simulink model "stumbler_simulation"  (R2024b)
settings: Solver=ode45  StartTime=0.0  StopTime=0.75  RelTol=1e-3  EnableMultiTasking=on
StopFcn:
  | plot_stumbler
settings Model: Creator=Marleen  LastModifiedBy=vijay
settings SolverCC: AlgebraicLoopSolver=TrustRegion
settings DataIOCC: LimitDataPoints=on  SaveFormat=Array  SignalLoggingSaveFormat=ModelDataLogs  ReturnWorkspaceOutputs=off
settings OptimizationCC: InitFltsAndDblsToZero=on  LifeSpan=inf
settings DebuggingCC: SaveWithParameterizedLinksMsg=none  UnderspecifiedInitializationDetection=Classic  MergeDetectMultiDrivingBlocksExec=none  SignalResolutionControl=TryResolveAllWithWarning  SolverPrmCheckMsg=warning  MultiTaskDSMMsg=warning  MultiTaskCondExecSysMsg=none  FcnCallInpInsideContextMsg=warning  UnconnectedInputMsg=warning  UnconnectedOutputMsg=warning  UnconnectedLineMsg=warning  SFUnexpectedBacktrackingDiag=warning  SFNoUnconditionalDefaultTransitionDiag=warning  SFExecutionAtInitializationDiag=none  ArithmeticOperatorsInVariantConditions=warning
settings HardwareCC: ProdBitPerPointer=32  ProdBitPerSizeT=32  ProdBitPerPtrDiffT=32  ProdLargestAtomicFloat=None  ProdIntDivRoundTo=Undefined  ProdEndianess=Unspecified  ProdWordSize=32  ProdHWDeviceType=32-bit Generic
settings ModelReferenceCC: EnableRefExpFcnMdlSchedulingChecks=on  PropagateSignalLabelsOutOfModel=off
settings SFSimCC: SimUseLocalCustomCode=off  CustomCodeUndefinedFunction=UseInterfaceOnly
settings RTWCC: RTWUseLocalCustomCode=off  GPUComputeCapability=3.5
settings CodeAppCC: StateflowObjectComments=on
settings GRTTargetCC: TargetFcnLib=ansi_tfl_tmw.mat  TargetLangStandard=C89/C90 (ANSI)  CombineOutputUpdateFcns=off  GRTInterface=on
settings ConfigComp: CovMetricSettings=dw  CovSaveCumulativeToWorkspaceVar=on  CovSaveSingleToWorkspaceVar=on  CovExternalEMLEnable=off

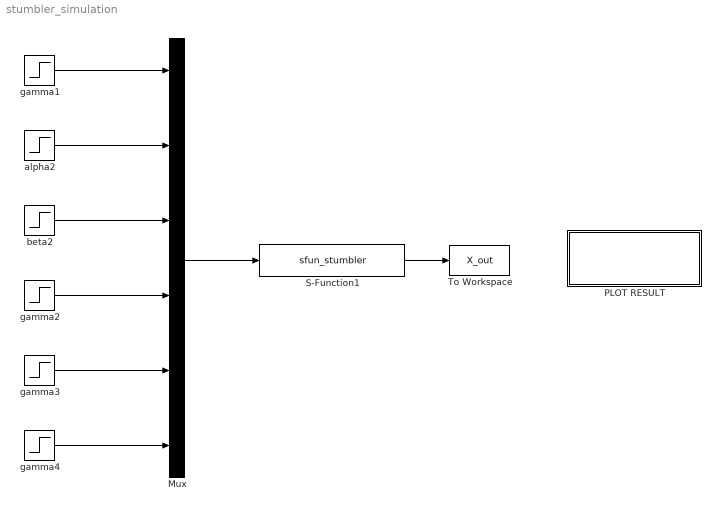
== system stumbler_simulation ==
  Mux : Mux  Inputs=6
  PLOT RESULT : Subsystem
      settings: OpenFcn=plot_stumbler
      mask Display: disp('DoubleClick to Animate')
  S-Function1 : S-Function  FunctionName=sfun_stumbler  SFunctionDeploymentMode=off  EnableBusSupport=off
  To Workspace : ToWorkspace  VariableName=X_out  SaveFormat=Structure With Time  SampleTime=0.01
  alpha2 : Step  Time=0  After=0  SampleTime=0
  beta2 : Step  Time=0  After=0  SampleTime=0
  gamma1 : Step  Time=0  After=0  SampleTime=0
  gamma2 : Step  Time=0  Before=3  After=-2  SampleTime=0
  gamma3 : Step  Time=0.15  Before=-5  SampleTime=0
  gamma4 : Step  Time=0  Before=1  After=2  SampleTime=0
  wires:
  S-Function1/1 -> To Workspace/1
  Mux/1 -> S-Function1/1
  gamma1/1 -> Mux/1
  alpha2/1 -> Mux/2
  beta2/1 -> Mux/3
  gamma2/1 -> Mux/4
  gamma3/1 -> Mux/5
  gamma4/1 -> Mux/6

== system stumbler_simulation/PLOT RESULT ==
